simulink model "pendu_vesc_modified"  (R2020a)
settings: Solver=FixedStepAuto  StartTime=0.0  StopTime=inf  RelTol=1e-3  EnableMultiTasking=on
model workspace (MAT data in the model file):
  Da = 2
  Du = 1
  H = 60
  J = 1
  K = 1
  M = {[0 0 3.14159265359 3.14159265359 -0.00627152337538 -0.789224693015 3.14032159952 3.14510265194 -0.41418344751 -0.875105999538 3.14549312601 3.14483529365 ... (244 elements, 4x61)]; []; []; []; []; []; []; []; []; []; []; []; []; []; []; []; []; []; []; []}
  N = 20
  S0 = [0.01  0  0  0; 0  0.01  0  0; 0  0  0.0001  0; 0  0  0  0.0001]
  S0Sim = [0.01  0  0  0; 0  0.01  0  0; 0  0  0.0001  0; 0  0  0  0.0001]
  Sig = Simulink.Signal
  Sig.DataType = 'auto'
  Sig.Dimensions = -1
  Sig.DimensionsMode = 'auto'
  Sig.Complexity = 'auto'
  Sig.SampleTime = -1
  Sig.SamplingMode = 'auto'
  Sig1 = Simulink.Signal
  Sig1.DataType = 'auto'
  Sig1.Dimensions = -1
  Sig1.DimensionsMode = 'auto'
  Sig1.Complexity = 'auto'
  Sig1.SampleTime = -1
  Sig1.SamplingMode = 'auto'
  Sigma = {[0.01 0 0 0 0 0.01 0 0 0 0 0.0001 0 ... (976 elements, 4x4x61)]; []; []; []; []; []; []; []; []; []; []; []; []; []; []; []; []; []; []; []}
  T = 3
  Xh = [3.23195665748  2.3666318046  2.58972132538  5.53764714904; 2.09576255698  2.42554352774  2.39370565159  5.08826507102; -0.136551314425  0.153414508771  -1.97475222314  -0.0826517468618; -0.588254405024  1.15994939546  1.22077212441  0.538962693011; -0.201907649817  0.45444453272  3.55830068563  -1.77726532542; 2.18567618171  2.31058191083  2.44494446055  1.91925708421; -3.25197677698  -0.937077299191  -5.7106587425  -4.30227247488; 1.14254532077  0.812469463157  1.11845994865  0.765773075836; -1.68859776393  -1.44002251202  -5.20580572667  0.202688714778]
  angi = [3 4]
  augi = []
  basename = 'pendubot_'
  cc = [0  0  0  0; 0  0  0  0; -9.9995000125e-05  -1.22458556834e-20  0  0; 0  0  -9.9995000125e-05  -1.22458556834e-20]
  cost.fcn : function handle (value not decoded)
  cost.gamma = 1
  cost.p = [0.5 0.5]
  cost.width = 0.25
  cost.expl = 0
  cost.angle = [3 4]
  cost.target = [0; 0; 0; 0]
  difi = [1 2 3 4]
  dt = 0.05
  dyni = [1 2 5 6 7 8]
  dynmodel.fcn : function handle (value not decoded)
  dynmodel.train : function handle (value not decoded)
  dynmodel.induce = []
  dynmodel.inputs = [0.0306796157577 -0.0230097118183 -0.0230097118183 -0.27412822575 0.0873506184902 1.75503381101 1.22816627149 -0.676608032868 -1.33717744439 -2.33662132144 -2.60950904676 -2.36326465025 ... (756 elements, 108x7)]
  dynmodel.targets = [-0.053689327576 0 -0.251118513931 0.36147884424 1.66768319252 -0.52686753952 -1.90477430435 -0.660569411519 -0.999443877058 -0.272887725314 0.246244396504 1.79597511908 ... (432 elements, 108x4)]
  dynmodel.hyp = [3.23195665748  2.3666318046  2.58972132538  5.53764714904; 2.09576255698  2.42554352774  2.39370565159  5.08826507102; -0.136551314425  0.153414508771  -1.97475222314  -0.0826517468618; -0.588254405024  1.15994939546  1.22077212441  0.538962693011; -0.201907649817  0.45444453272  3.55830068563  -1.77726532542; 2.18567618171  2.31058191083  2.44494446055  1.91925708421; -3.25197677698  -0.937077299191  -5.7106587425  -4.30227247488; 1.14254532077  0.812469463157  1.11845994865  0.765773075836; -1.68859776393  -1.44002251202  -5.20580572667  0.202688714778]
  dyno = [1 2 3 4]
  fX3 = [57.5848751283 57.5848706735 57.584870567 57.5848705445 57.584869604 57.5848692003 57.5848690287 57.584868717 57.5848685976 57.5848685293 57.5848683991 57.5848682957 ... (151 elements, 151x1)]
  fantasy.mean = {[1 0.96654934359 0.960216156363 0.959677125864 0.959626206088 0.959621245001 0.959620752058 0.95962070215 0.959620697005 0.959620696465 0.959620696408 0.959620696402 0.959620696401 0.959620696401 0.959620696401 0.959620696401 0.959620696401 0.959620696401 0.959620696401 0.959620696401 0.959620696401 0.959620696401 0.959620696401 0.959620696401 0.959620696401 0.959620696401 0.959620696401 0.959620696401 0.959620696401 0.959620696401 0.959620696401 0.959620696401 0.959620696401 0.959620696401 0.959620696401 0.959620696401 0.959620696401 0.959620696401 0.959620696401 0.959620696401 0.959620696401 0.959620696401 0.959620696401 0.959620696401 0.959620696401 0.959620696401 0.959620696401 0.959620696401 0.959620696401 0.959620696401 0.959620696401 0.959620696401 0.959620696401 0.959620696401 0.959620696401 0.959620696401 0.959620696401 0.959620696401 0.959620696401 0.959620696401 0.959620696401], [], [], [], [], [], [], [], [], [], [], [], [], [], [], [], [], [], [], []}
  fantasy.std = {[0 0.118697886946 0.129956951664 0.130859326759 0.130944136654 0.130952395646 0.130953216236 0.130953299316 0.130953307881 0.130953308779 0.130953308874 0.130953308885 0.130953308886 0.130953308886 0.130953308886 0.130953308886 0.130953308886 0.130953308886 0.130953308886 0.130953308886 0.130953308886 0.130953308886 0.130953308886 0.130953308886 0.130953308886 0.130953308886 0.130953308886 0.130953308886 0.130953308886 0.130953308886 0.130953308886 0.130953308886 0.130953308886 0.130953308886 0.130953308886 0.130953308886 0.130953308886 0.130953308886 0.130953308886 0.130953308886 0.130953308886 0.130953308886 0.130953308886 0.130953308886 0.130953308886 0.130953308886 0.130953308886 0.130953308886 0.130953308886 0.130953308886 0.130953308886 0.130953308886 0.130953308886 0.130953308886 0.130953308886 0.130953308886 0.130953308886 0.130953308886 0.130953308886 0.130953308886 0.130953308886], [], [], [], [], [], [], [], [], [], [], [], [], [], [], [], [], [], [], []}
  i = 108
  j = 1
  mm = [0; 0; 3.14159265359; 3.14159265359; 1.22458556834e-16; -0.99995000125; 1.22458556834e-16; -0.99995000125]
  mu0 = [0; 0; 3.14159265359; 3.14159265359]
  mu0Sim = [0; 0; 3.14159265359; 3.14159265359]
  nc = 200
  odei = [1 2 3 4]
  opt.length = 150
  opt.MFEPLS = 20
  opt.verbosity = 1
  opt.method = 'BFGS'
  opt.fh = 1
  plant.dynamics : function handle (value not decoded)
  plant.noise = [0.0001  0  0  0; 0  0.0001  0  0; 0  0  0.0001  0; 0  0  0  0.0001]
  plant.dt = 0.05
  plant.ctrl : function handle (value not decoded)
  plant.odei = [1 2 3 4]
  plant.augi = []
  plant.angi = [3 4]
  plant.poli = [1 2 5 6 7 8]
  plant.dyno = [1 2 3 4]
  plant.dyni = [1 2 5 6 7 8]
  plant.difi = [1 2 3 4]
  plant.prop : function handle (value not decoded)
  plotting.verbosity = 1
  poli = [1 2 5 6 7 8]
  policy.fcn : function handle (value not decoded)
  policy.maxU = 3.5
  policy.p.inputs = [0.102572533398 0.209073779707 -0.0880163417462 0.0820849246411 -0.16346836167 -0.0378904445118 0.0309050415451 0.156557665361 0.0211361233155 -0.112243464011 -0.0637123277078 0.0761350182082 ... (1200 elements, 200x6)]
  policy.p.targets = [-0.0683206925151 0.0784477829767 -0.0270909739403 0.014497250572 0.20614993253 0.0211015325481 -0.0369305155107 0.0894433826752 -0.0127436267208 0.0448484706497 -0.00865317778938 -0.0188315455954 ... (200 elements, 200x1)]
  policy.p.hyp = [-0.0231632148156; -0.0227454895619; -0.375748702272; -0.385515894844; -0.391084497867; -0.396204678577; 0; -4.60517018599]
  rd = '../../'
  realCost = {[], [], [], [], [], [], [], [], [], [], [], [], [], [], [], [], [], [], [], []}
  record_data = [3.14159265359 -3.1396751776 0.0306796157577 0 0 3.14159265359 -3.1408256632 -0.0230097118183 0 0.0167798938511 3.14159265359 3.14120915839 ... (545 elements, 5x109)]
  s = [3.99154064865; -6.40884909322; 3.07813248092; -2.1607954049; 0.0634175868444; -0.997987078914; -0.830941192004; -0.556360256876]
  sa = [0.0634175868444; -0.997987078914; -0.830941192004; -0.556360256876]
  ss = [0.01  0  0  0  0  0  0  0; 0  0.01  0  0  0  0  0  0; 0  0  0.0001  0  -9.9995000125e-05  -1.22458556834e-20  0  0; 0  0  0  0.0001  0  0  -9.9995000125e-05  -1.22458556834e-20; 0  0  -9.9995000125e-05  0  9.99900006666e-05  1.22446311641e-20  0  0; 0  0  -1.22458556834e-20  0  1.22446311641e-20  4.99950003618e-09  0  0; 0  0  0  -9.9995000125e-05  0  0  9.99900006666e-05  1.22446311641e-20; 0  0  0  -1.22458556834e-20  0  0  1.22446311641e-20  4.99950003618e-09]
  trainOpt = [200 200]
  x = [0.0306796157577 -0.0230097118183 -0.0230097118183 -0.27412822575 0.0873506184902 1.75503381101 1.22816627149 -0.676608032868 -1.33717744439 -2.33662132144 -2.60950904676 -2.36326465025 ... (972 elements, 108x9)]
  x_ = [3.14159265359 3.14159265359 3.14159265359 -3.11771653557 -3.0819023985 -3.13719441642 3.01718558664 2.86638914992 2.73318560862 2.6734953269 2.7155927132 2.87392898507 ... (540 elements, 108x5)]
  xaug = [0.0306796157577 -0.0230097118183 -0.0230097118183 -0.27412822575 0.0873506184902 1.75503381101 1.22816627149 -0.676608032868 -1.33717744439 -2.33662132144 -2.60950904676 -2.36326465025 ... (864 elements, 108x8)]
  y = [-0.0230097118183 -0.0230097118183 -0.27412822575 0.0873506184902 1.75503381101 1.22816627149 -0.676608032868 -1.33717744439 -2.33662132144 -2.60950904676 -2.36326465025 -0.567289531178 ... (432 elements, 108x4)]
  y_ = [3.14159265359 3.14159265359 -3.11771653557 -3.0819023985 -3.13719441642 3.01718558664 2.86638914992 2.73318560862 2.6734953269 2.7155927132 2.87392898507 3.11017672705 ... (432 elements, 108x4)]
undefined symbols (not defined in the file or in its folder): DiscIntNeverNeededParam
libraries: eeGeneralControl x3, cm_custom x2, simulink x1
(part 1 of 2)
settings Model: SimulationMode=external  OrderedModelArguments=off  Creator=Ng Wee Shen  LastModifiedBy=BMT Group
settings SolverCC: PositivePriorityOrder=on  AutoInsertRateTranBlk=on
settings DataIOCC: ReturnWorkspaceOutputs=off
settings OptimizationCC: EnhancedBackFolding=on  PassReuseOutputArgsAs=Individual arguments  MaxStackSize=64  OptimizeBlockOrder=speed  DifferentSizesBufferReuse=on  EfficientTunableParamExpr=on
settings DebuggingCC: TimeAdjustmentMsg=warning  SingleTaskRateTransMsg=warning  ParameterTunabilityLossMsg=error  SFcnCompatibilityMsg=warning  UnderSpecifiedDimensionMsg=error  ArithmeticOperatorsInVariantConditions=warning
settings HardwareCC: ProdBitPerPointer=32  ProdBitPerSizeT=32  ProdBitPerPtrDiffT=32  ProdLargestAtomicInteger=Long  ProdLargestAtomicFloat=Double  ProdWordSize=32  ProdHWDeviceType=ARM Compatible->ARM Cortex
settings SFSimCC: MATLABDynamicMemAlloc=off  CustomCodeUndefinedFunction=UseInterfaceOnly
settings RTWCC: SystemTargetFile=ert.tlc  HardwareBoard=Raspberry Pi  TemplateMakefile=ert_default_tmf  Toolchain=GNU GCC Raspberry Pi  BuildConfiguration=Specify  IncludeHyperlinkInReport=on  TargetLang=C++
settings CodeAppCC: ForceParamTrailComments=on  IgnoreCustomStorageClasses=off  OperatorAnnotations=on  SimulinkDataObjDesc=on  SFDataObjDesc=on  InsertBlockDesc=on
settings ERTTargetCC: TargetLangStandard=C++03 (ISO)  SupportContinuousTime=on  SupportVariableSizeSignals=on  ExtMode=on  ExtModeMexArgs='192.168.0.173' 1 17725

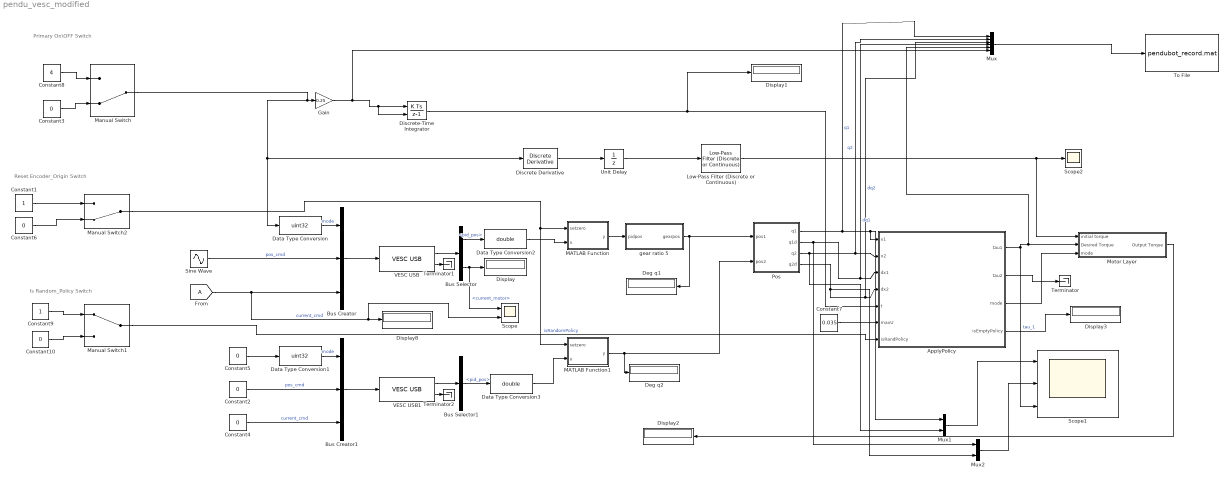
== system pendu_vesc_modified ==
  note: Primary On\OFF Switch
  note: Reset Encoder_Origin Switch
  note: Is Random_Policy Switch
  ApplyPolicy : MATLAB Function  TreatAsAtomicUnit=on
  Bus Creator : BusCreator  Inputs=3
  Bus Creator1 : BusCreator  Inputs=3
  Bus Selector : BusSelector  OutputSignals=pid_pos,current_motor
  Bus Selector1 : BusSelector  OutputSignals=pid_pos
  Constant1 : Constant
  Constant{2..6,10} (6 alike) : Constant  Value=0
  Constant7 : Constant  Value=0.035
  Constant8 : Constant  Value=4
  Constant9 : Constant
  Data Type Conversion : DataTypeConversion  OutDataTypeStr=uint32
  Data Type Conversion1 : DataTypeConversion  OutDataTypeStr=uint32
  Data Type Conversion2 : DataTypeConversion  OutDataTypeStr=double
  Data Type Conversion3 : DataTypeConversion  OutDataTypeStr=double
  Deg q1 : Display
  Deg q2 : Display
  Discrete Derivative : simulink/Discrete/Discrete Derivative  gainval=1.0  ICPrevScaledInput=0.0  OutMin=[]  OutMax=[]  OutDataType=fixdt(1, 16)  OutScaling=2^-10  DoSatur=off
  Discrete-Time Integrator : DiscreteIntegrator  ExternalReset=falling  SampleTime=-1  ICPrevOutput=DiscIntNeverNeededParam  ICPrevScaledInput=DiscIntNeverNeededParam
  Display{,1..3,8} (5 alike) : Display
  Gain : Gain  Gain=0.25
  Low-Pass Filter (Discrete or Continuous) : eeGeneralControl/Low-Pass Filter (Discrete or Continuous)  K=-1  T=0.025  B=0.05  A=-0.05  init_option=Inherited from block input  x0=0  Ts=-1
  MATLAB Function : MATLAB Function  TreatAsAtomicUnit=on
  MATLAB Function1 : MATLAB Function  TreatAsAtomicUnit=on
  Manual Switch : ManualSwitch  CurrentSetting=0
  Manual Switch1 : ManualSwitch
  Manual Switch2 : ManualSwitch  CurrentSetting=0
  Motor Layer : Subsystem
  Mux : Mux  Inputs=6
  Mux1 : Mux  Inputs=2
  Mux2 : Mux  Inputs=2
  Pos : Subsystem
  Scope : Scope  NumInputPorts=2
  Scope1 : Scope  NumInputPorts=3
  Scope2 : Scope
  Sine Wave : Sin  Amplitude=150  Bias=10  SampleTime=0
  Terminator : Terminator
  Terminator1 : Terminator
  Terminator2 : Terminator
  To File : ToFile  Filename=pendubot_record.mat  MatrixName=record_data
  Unit Delay : UnitDelay  SampleTime=-1  HasFrameUpgradeWarning=on
  VESC USB : cm_custom/VESC USB  PAR_VESC_DEV='/dev/VESC2'  POS_KP=0.03  POS_KI=0  POS_KD=0.0004  POS_KD_FIL=0.2  POS_DIV=1  CURR_MAX=6  CURR_MIN=-6  CURR_IN_MAX=99  CURR_IN_MIN=-60  CURR_ABS_MAX=130  PAR_SMPLT=0.001
      settings: SourceProductName=cm custom
  VESC USB1 : cm_custom/VESC USB  PAR_VESC_DEV='/dev/VESC1'  POS_KP=0.001  POS_KI=0  POS_KD=0.001  POS_KD_FIL=0.2  POS_DIV=1  CURR_MAX=20  CURR_MIN=-20  CURR_IN_MAX=20  CURR_IN_MIN=-20  CURR_ABS_MAX=20  PAR_SMPLT=0.001
      settings: SourceProductName=cm custom
  gear ratio 5 : Subsystem
  wires:
  Bus Creator/1 -> VESC USB/1
  VESC USB/1 -> Bus Selector/1
  VESC USB/2 -> Terminator1/1
  Data Type Conversion/1 -> Bus Creator/1  "mode"
  Bus Selector/2 -> Display/1, Scope/1  "<current_motor>"
  Bus Selector/1 -> Data Type Conversion2/1  "<pid_pos>"
  Constant3/1 -> Manual Switch/2
  Sine Wave/1 -> Bus Creator/2  "pos_cmd"
  [A] -> Scope/2, Display8/1, Bus Creator/3  "current_cmd"
  Constant4/1 -> Bus Creator1/3  "current_cmd"
  Data Type Conversion1/1 -> Bus Creator1/1  "mode"
  Constant2/1 -> Bus Creator1/2  "pos_cmd"
  Bus Creator1/1 -> VESC USB1/1
  Constant5/1 -> Data Type Conversion1/1
  Bus Selector1/1 -> Data Type Conversion3/1  "<pid_pos>"
  VESC USB1/1 -> Bus Selector1/1
  VESC USB1/2 -> Terminator2/1
  Pos/1(q1) -> Mux1/1, ApplyPolicy/1(x1), Mux/1  "q1"
  Pos/2(q1d) -> Mux/4, ApplyPolicy/3(dx1), Mux2/1  "dq1"
  Pos/4(q2d) -> Mux2/2, Mux/3, ApplyPolicy/4(dx2)  "dq2"
  Motor Layer/1(Output Torque) -> Display2/1
  ApplyPolicy/3(mode) -> Motor Layer/3(" mode ")
  Data Type Conversion2/1 -> MATLAB Function/2(u)
  MATLAB Function1/1(y) -> Pos/2(pos2), Deg q2/1
  Data Type Conversion3/1 -> MATLAB Function1/2(u)
  Constant1/1 -> Manual Switch2/1
  Constant6/1 -> Manual Switch2/2
  Manual Switch2/1 -> MATLAB Function1/1(setzero), MATLAB Function/1(setzero)
  Pos/3(q2) -> Mux1/2, Mux/2, ApplyPolicy/2(x2)  "q2"
  MATLAB Function/1(y) -> gear ratio 5/1(pidpos)
  gear ratio 5/1(gearpos) -> Pos/1(pos1), Deg q1/1
  Manual Switch/1 -> Data Type Conversion/1, Discrete Derivative/1, Gain/1
  ApplyPolicy/1(tau1) -> Mux/5, Motor Layer/2(Desired Torque), Scope1/3  "tau_1"
  Unit Delay/1 -> Low-Pass Filter (Discrete or Continuous)/1
  Low-Pass Filter (Discrete or Continuous)/1 -> Motor Layer/1(initial torque), Scope2/1
  ApplyPolicy/2(tau2) -> Terminator/1
  Discrete Derivative/1 -> Unit Delay/1
  Discrete-Time Integrator/1 -> ApplyPolicy/5(t), Display1/1
  Constant7/1 -> ApplyPolicy/6(maxU)
  Mux/1 -> To File/1
  Constant8/1 -> Manual Switch/1
  Gain/1 -> Mux/6, Discrete-Time Integrator/1, Discrete-Time Integrator/2
  Constant9/1 -> Manual Switch1/1
  Constant10/1 -> Manual Switch1/2
  Manual Switch1/1 -> ApplyPolicy/7(isRandPolicy)  "isRandomPolicy"
  Mux1/1 -> Scope1/1
  Mux2/1 -> Scope1/2
  ApplyPolicy/4(isEmptyPolicy) -> Display3/1
